simulink library "PMPSpoolingController_ul"  (R2018b)
settings: Solver=VariableStepAuto  StartTime=0.0  StopTime=10.0  RelTol=1e-3
undefined symbols (not defined in the file or in its folder): guess, kd_iter, ki_iter, kp_iter, pathCtrl, speedRange, Ten
settings Model: Creator=James Reed  LastModifiedBy=jldanie5

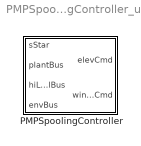
== system PMPSpoolingController_ul ==
  PMPSpoolingController : Subsystem

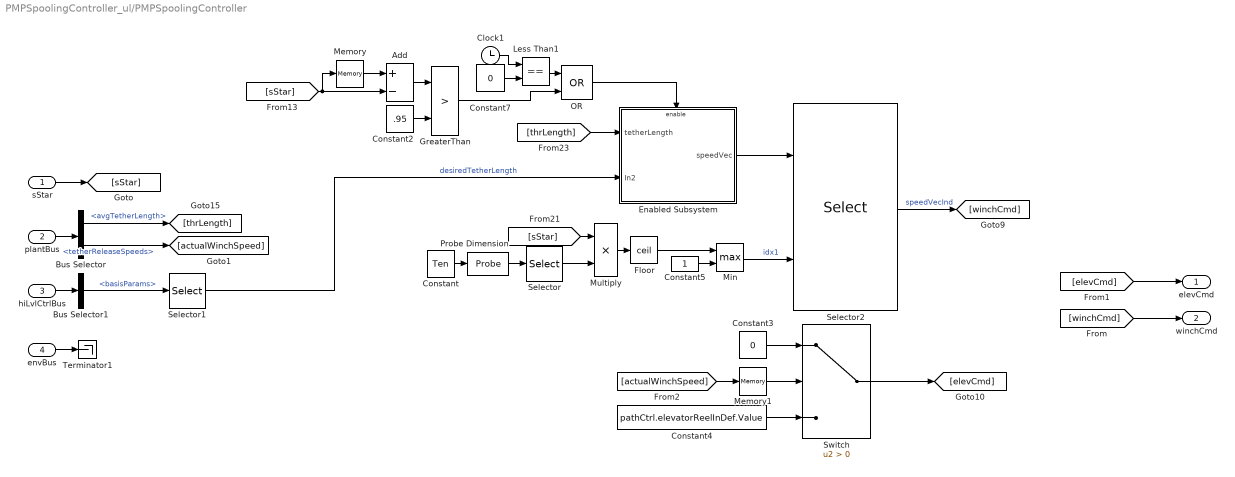
== system PMPSpoolingController_ul/PMPSpoolingController ==
  "sStar " : Inport
  plantBus : Inport  Port=2  OutDataTypeStr=Bus: plantBus
  hiLvlCtrlBus : Inport  Port=3  OutDataTypeStr=Bus: hiLvlCtrlBus
  envBus : Inport  Port=4  OutDataTypeStr=Bus: envBus
  Add : Sum  Inputs=+-
  Bus Selector : BusSelector  OutputSignals=avgTetherLength,tetherReleaseSpeeds
  Bus Selector1 : BusSelector  OutputSignals=basisParams
  Clock1 : Clock
  Constant : Constant  Value=Ten
  Constant2 : Constant  Value=.95
  Constant3 : Constant  Value=0
  Constant4 : Constant  Value=pathCtrl.elevatorReelInDef.Value
  Constant5 : Constant
  Constant7 : Constant  Value=0
  Enabled Subsystem : Subsystem  TreatAsAtomicUnit=on
  Floor : Rounding  Operator=ceil
  GreaterThan : RelationalOperator  Operator=>  OutDataTypeStr=boolean  RndMeth=Simplest
  Less Than1 : RelationalOperator  Operator===  OutDataTypeStr=boolean  RndMeth=Simplest
  Memory : Memory  InitialCondition=pathCtrl.initPathVar.Value
  Memory1 : Memory
  Min : MinMax  Function=max  Inputs=2
  Multiply : Product
  OR : Logic  Operator=OR  IconShape=distinctive  AllPortsSameDT=off  OutDataTypeStr=boolean
  Probe Dimension : Probe  ProbeWidth=off  ProbeSampleTime=off  ProbeComplexSignal=off  ProbeSignalDimensions=on
  Selector : Selector  InputPortWidth=2  IndexOptions=Index vector (dialog)  Indices=1  OutputSizes=1
  Selector1 : Selector  IndexOptions=Index vector (dialog)  Indices=5  OutputSizes=1
  Selector2 : Selector  InputPortWidth=TenWidth  IndexOptions=Index vector (port)  Indices=[1 3]  OutputSizes=1
  Switch : Switch  Criteria=u2 > Threshold
  Terminator1 : Terminator
  elevCmd : Outport
  "winchCmd " : Outport  Port=2
  wires:
  [winchCmd] -> "winchCmd "/1
  hiLvlCtrlBus/1 -> Bus Selector1/1
  [elevCmd] -> elevCmd/1
  "sStar "/1 -> [sStar]
  plantBus/1 -> Bus Selector/1
  envBus/1 -> Terminator1/1
  OR/1 -> Enabled Subsystem/Enable
  Constant7/1 -> Less Than1/2
  [sStar] -> Memory/1, Add/2
  Less Than1/1 -> OR/1
  GreaterThan/1 -> OR/2
  Multiply/1 -> Floor/1
  Add/1 -> GreaterThan/1
  Floor/1 -> Min/1
  Min/1 -> Selector2/2  "idx1"
  Switch/1 -> [elevCmd]
  Constant5/1 -> Min/2
  Constant4/1 -> Switch/3
  Memory/1 -> Add/1
  Selector/1 -> Multiply/2
  Constant2/1 -> GreaterThan/2
  Selector2/1 -> [winchCmd]  "speedVecInd"
  Constant3/1 -> Switch/1
  [thrLength] -> Enabled Subsystem/1(tetherLength)
  [sStar] -> Multiply/1
  Enabled Subsystem/1(speedVec) -> Selector2/1
  Clock1/1 -> Less Than1/1
  Bus Selector/1 -> [thrLength]  "<avgTetherLength>"
  Constant/1 -> Probe Dimension/1
  Probe Dimension/1 -> Selector/1
  Bus Selector1/1 -> Selector1/1  "<basisParams>"
  Selector1/1 -> Enabled Subsystem/2(In2)  "desiredTetherLength"
  [actualWinchSpeed] -> Memory1/1
  Bus Selector/2 -> [actualWinchSpeed]  "<tetherReleaseSpeeds>"
  Memory1/1 -> Switch/2

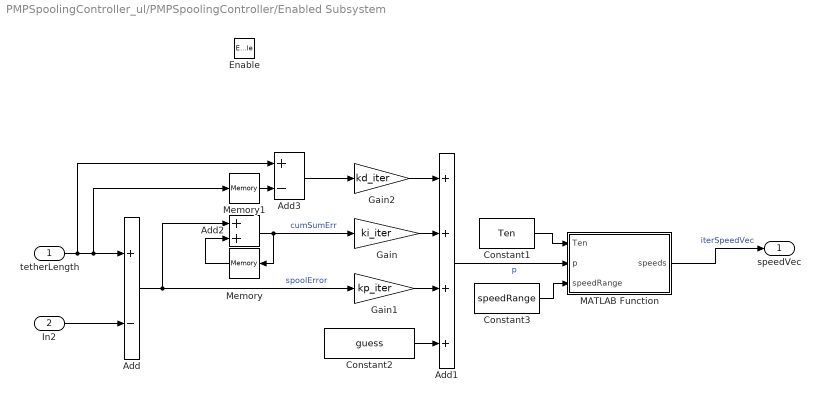
== system PMPSpoolingController_ul/PMPSpoolingController/Enabled Subsystem ==
  tetherLength : Inport
  In2 : Inport  Port=2
  Enable : EnablePort
  Add : Sum  Inputs=+-
  Add1 : Sum  Inputs=++++
  Add2 : Sum
  Add3 : Sum  Inputs=+-
  Constant1 : Constant  Value=Ten
  Constant2 : Constant  Value=guess
  Constant3 : Constant  Value=speedRange
  Gain : Gain  Gain=ki_iter
  Gain1 : Gain  Gain=kp_iter
  Gain2 : Gain  Gain=kd_iter
  MATLAB Function : MATLAB Function  TreatAsAtomicUnit=on
  Memory : Memory
  Memory1 : Memory
  speedVec : Outport
  wires:
  Gain2/1 -> Add1/1
  Add3/1 -> Gain2/1
  Memory1/1 -> Add3/2
  In2/1 -> Add/2
  tetherLength/1 -> Add/1, Memory1/1, Add3/1
  Constant2/1 -> Add1/4
  Memory/1 -> Add2/2
  Constant1/1 -> MATLAB Function/1(Ten)
  Add1/1 -> MATLAB Function/2(p)  "p"
  MATLAB Function/1(speeds) -> speedVec/1  "iterSpeedVec"
  Gain1/1 -> Add1/3
  Gain/1 -> Add1/2
  Add2/1 -> Gain/1, Memory/1  "cumSumErr"
  Add/1 -> Gain1/1, Add2/1  "spoolError"
  Constant3/1 -> MATLAB Function/3(speedRange)

== matlab function PMPSpoolingController_ul/PMPSpoolingController/Enabled Subsystem/MATLAB Function ==
  data: Ten input; speeds output; p input; speedRange input
function speeds = fcn(Ten, p, speedRange)
xopts=linspace(speedRange(1),speedRange(2),max(size(Ten)));
n=1000;
% speeds = zeros(2*max(size(Ten)),1);
speeds = zeros(n,1);
% for ii = 1:2*max(size(Ten))
for ii = 1:n
    iidbl=(1000/n)*ii;
    %     hamil = @(x) (p-Ten(ii,xopts==x)).*x;
    perc=iidbl-floor(iidbl);
    currTen=((1-perc)*Ten(max(floor(iidbl),1),:)) + (perc*Ten(ceil(iidbl),:));
    hamil = @(x) (p-interp1(xopts,currTen,x)).*x;
    [~,bestind]=min(hamil(xopts));
    bestx=xopts(bestind);
    
    step=xopts(2)-xopts(1);
    lbnd = max(xopts(1),bestx-step);
    rbnd = min(xopts(end),bestx+step);
    tau = 1-.38197;
    for i=1:5
        x1=((1-tau)*rbnd)+(tau*lbnd);
        x2=((1-tau)*lbnd)+(tau*rbnd);
        f1=hamil(x1);
        f2=hamil(x2);
        if f1>=f2
            lbnd=x1;
        else
            rbnd=x2;
        end
    end
    bestx=(lbnd+rbnd)/2;
    speeds(ii)=bestx;
end
